simulink subsystem "InsulatedPipe"  (R2022b)
settings: Solver=VariableStepAuto  StartTime=0.0  StopTime=10.0  RelTol=1e-3
model mask{D=0, dh=0}
  mask prompts: D "Diameter"; dh "Elevation Change"
undefined symbols (not defined in the file or in its folder): Dpipe
libraries: fl_lib x3
settings Model: Creator=vboutrou  LastModifiedBy=vboutrou

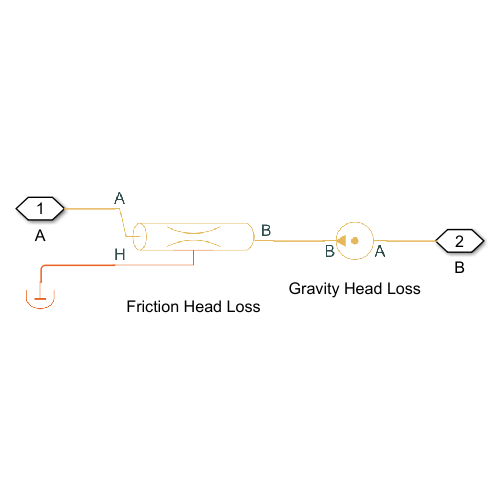
[thumbnail: Simulink's stored preview of the top-level diagram]
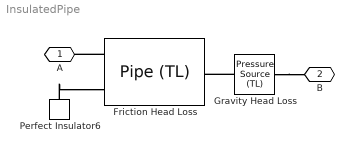
== system InsulatedPipe ==
  Friction Head Loss : fl_lib/Thermal Liquid/Elements/Pipe (TL)  length=1 m  area=pi*D^2/4 in^2  Dh=D in  length_add=1 m  roughness=15e-6 m  Re_lam=2000  Re_tur=4000  shape_factor=64  Nu_lam=3.66  dynamic_compressibility=simscape.enum.onoff.on  inertia=simscape.enum.onoff.off  p0=0.101325 MPa  T0=85 degC  mdot0=0 kg/s
  Gravity Head Loss : fl_lib/Thermal Liquid/Sources/Pressure Source (TL)  commanded_pressure=dh/9.81 bar  area=pi*Dpipe^2/4 in^2
      settings: InternalSimscapePortConfiguration="{\"Bottom\":[],\"Left\":[{\"id\":\"A\",\"label\":\"A\",\"type\":\"foundation.thermal_liquid.thermal_liquid\"}],\"Right\":[{\"id\":\"B\",\"label\":\"B\",\"type\":\"foundation.thermal_liquid.thermal_liquid\"}],\"Top\":[]}"
  Perfect Insulator6 : fl_lib/Thermal/Thermal Elements/Perfect Insulator  T_specify=off  T_priority=None  T=293.15 K  T_nominal_specify=off  T_nominal_unit=K  T_nominal_value=1
  A : PMIOPort  Side=Left
  B : PMIOPort  Port=2  Side=Right
  connections:
  Gravity Head Loss/LConn1 -- B/RConn1
  Friction Head Loss/LConn1 -- A/RConn1
  Gravity Head Loss/RConn1 -- Friction Head Loss/RConn1
  Perfect Insulator6/LConn1 -- Friction Head Loss/LConn2
